simulink model "test"  (R2020a)
settings: Solver=ode8  StartTime=0.0  StopTime=10.0  RelTol=1e-3
settings Model: Creator=meagh  LastModifiedBy=meagh
settings RTWCC: Description=Generic Real-Time Target

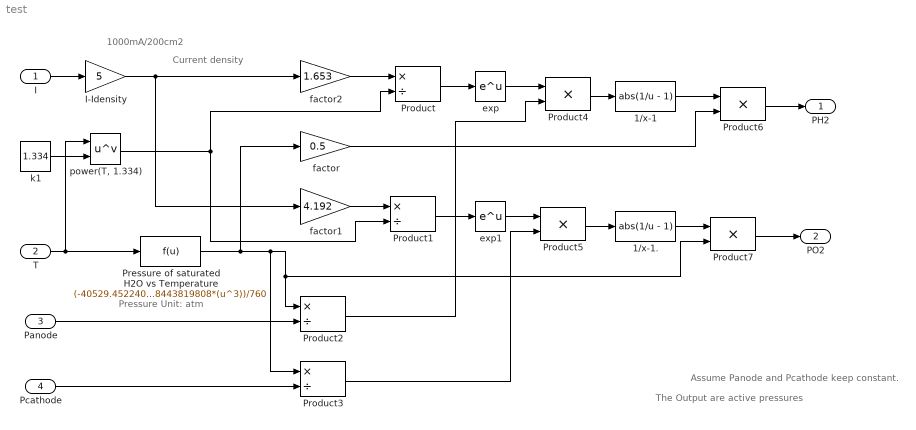
== system test ==
  note: Assume Panode and Pcathode keep constant.
  note: Pressure Unit: atm
  note: The Output are active pressures
  note: Current density
  note: 1000mA/200cm2
  I : Inport
  T : Inport  Port=2
  Panode : Inport  Port=3
  Pcathode : Inport  Port=4
  1/x-1 : Fcn  Expr=abs(1/u - 1)
  1/x-1. : Fcn  Expr=abs(1/u - 1)
  I-Idensity : Gain  Gain=5  SaturateOnIntegerOverflow=on  OutDataTypeStr=Inherit: Same as input  ParamDataTypeStr=Inherit: Same as input
  Pressure of saturated H2O vs Temperature : Fcn  Expr=(-40529.4522405347 + 401.94033912153*u-1.33430273535993*(u^2) + 0.00148378443819808*(u^3))/760
  Product{,1..3} (4 alike) : Product  Inputs=*/  SaturateOnIntegerOverflow=on  OutDataTypeStr=Inherit: Same as first input
  Product{4..7} (4 alike) : Product  SaturateOnIntegerOverflow=on  OutDataTypeStr=Inherit: Same as first input
  exp : Math  SignedPower=on  SaturateOnIntegerOverflow=on
  exp1 : Math  SignedPower=on  SaturateOnIntegerOverflow=on
  factor : Gain  Gain=0.5  SaturateOnIntegerOverflow=on  OutDataTypeStr=Inherit: Same as input  ParamDataTypeStr=Inherit: Same as input
  factor1 : Gain  Gain=4.192  SaturateOnIntegerOverflow=on  OutDataTypeStr=Inherit: Same as input  ParamDataTypeStr=Inherit: Same as input
  factor2 : Gain  Gain=1.653  SaturateOnIntegerOverflow=on  OutDataTypeStr=Inherit: Same as input  ParamDataTypeStr=Inherit: Same as input
  k1 : Constant  Value=1.334
  "power(T, 1.334)" : Math  Operator=pow  SignedPower=on  SaturateOnIntegerOverflow=on
  PH2 : Outport
  PO2 : Outport  Port=2
  wires:
  exp1/1 -> Product5/1
  Product3/1 -> Product5/2
  1/x-1./1 -> Product7/1
  factor/1 -> Product6/2
  I-Idensity/1 -> factor1/1, factor2/1
  Product6/1 -> PH2/1
  Product1/1 -> exp1/1
  Product2/1 -> Product4/2
  factor2/1 -> Product/1
  factor1/1 -> Product1/1
  Pcathode/1 -> Product3/2
  1/x-1/1 -> Product6/1
  Product4/1 -> 1/x-1/1
  Panode/1 -> Product2/2
  Product/1 -> exp/1
  exp/1 -> Product4/1
  T/1 -> "power(T, 1.334)"/1, Pressure of saturated H2O vs Temperature/1
  Pressure of saturated H2O vs Temperature/1 -> factor/1, Product3/1, Product2/1, Product7/2
  k1/1 -> "power(T, 1.334)"/2
  "power(T, 1.334)"/1 -> Product/2, Product1/2
  Product5/1 -> 1/x-1./1
  I/1 -> I-Idensity/1
  Product7/1 -> PO2/1
